simulink model "mVariantSubsystemConfig"  (R2019b)
settings: Solver=VariableStepAuto  StartTime=0.0  StopTime=10.0  RelTol=1e-3
settings Model: Creator=9bt  LastModifiedBy=4qz

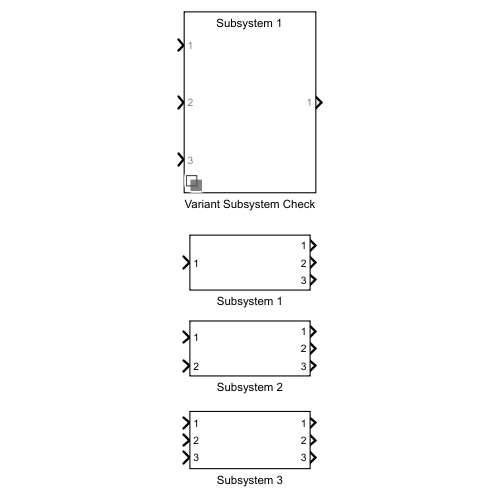
[thumbnail: Simulink's stored preview of the top-level diagram]
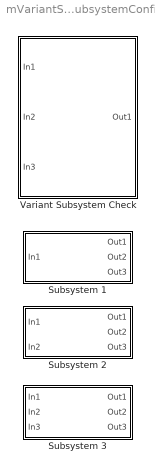
== system mVariantSubsystemConfig ==
  Subsystem 1 : Subsystem  VariantControl=Choice_1
  Subsystem 2 : Subsystem  VariantControl=Choice_2
  Subsystem 3 : Subsystem  VariantControl=Choice_3
  Variant Subsystem Check : Subsystem  Variant=on  VariantControlMode=label  LabelModeActiveChoice=Choice_1

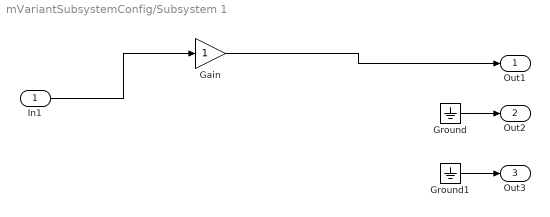
== system mVariantSubsystemConfig/Subsystem 1 ==
  In1 : Inport
  Gain : Gain
  Ground : Ground
  Ground1 : Ground
  Out1 : Outport
  Out2 : Outport  Port=2
  Out3 : Outport  Port=3
  wires:
  In1/1 -> Gain/1
  Gain/1 -> Out1/1
  Ground/1 -> Out2/1
  Ground1/1 -> Out3/1

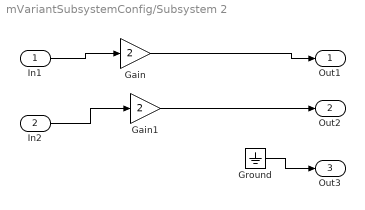
== system mVariantSubsystemConfig/Subsystem 2 ==
  In1 : Inport
  In2 : Inport  Port=2
  Gain : Gain  Gain=2
  Gain1 : Gain  Gain=2
  Ground : Ground
  Out1 : Outport
  Out2 : Outport  Port=2
  Out3 : Outport  Port=3
  wires:
  Gain1/1 -> Out2/1
  Gain/1 -> Out1/1
  In1/1 -> Gain/1
  In2/1 -> Gain1/1
  Ground/1 -> Out3/1

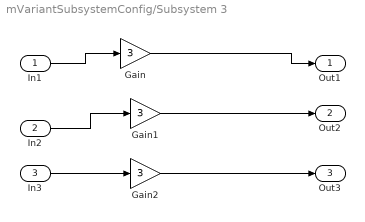
== system mVariantSubsystemConfig/Subsystem 3 ==
  In1 : Inport
  In2 : Inport  Port=2
  In3 : Inport  Port=3
  Gain : Gain  Gain=3
  Gain1 : Gain  Gain=3
  Gain2 : Gain  Gain=3
  Out1 : Outport
  Out2 : Outport  Port=2
  Out3 : Outport  Port=3
  wires:
  In2/1 -> Gain1/1
  Gain1/1 -> Out2/1
  Gain/1 -> Out1/1
  Gain2/1 -> Out3/1
  In1/1 -> Gain/1
  In3/1 -> Gain2/1

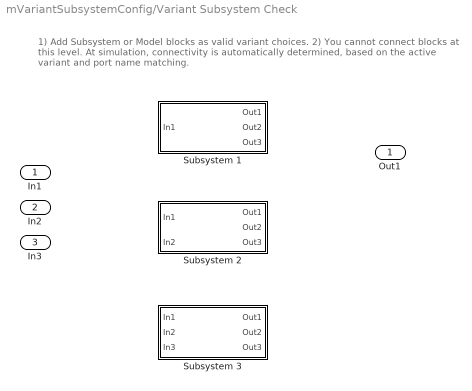
== system mVariantSubsystemConfig/Variant Subsystem Check ==
  note: 1) Add Subsystem or Model blocks as valid variant choices.
      | 2) You cannot connect blocks at this level. At simulation, connectivity is automatically
      | determined, based on the active variant and port name matching.
  In1 : Inport
  In2 : Inport  Port=2
  In3 : Inport  Port=3
  Subsystem 1 : Subsystem  VariantControl=Choice_1
  Subsystem 2 : Subsystem  VariantControl=Choice_2
  Subsystem 3 : Subsystem  VariantControl=Choice_3
  Out1 : Outport

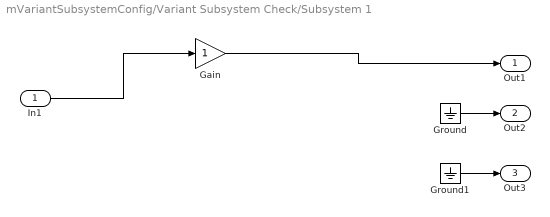
== system mVariantSubsystemConfig/Variant Subsystem Check/Subsystem 1 ==
  In1 : Inport
  Gain : Gain
  Ground : Ground
  Ground1 : Ground
  Out1 : Outport
  Out2 : Outport  Port=2
  Out3 : Outport  Port=3
  wires:
  In1/1 -> Gain/1
  Gain/1 -> Out1/1
  Ground/1 -> Out2/1
  Ground1/1 -> Out3/1

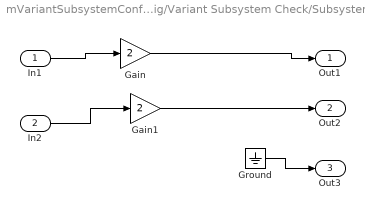
== system mVariantSubsystemConfig/Variant Subsystem Check/Subsystem 2 ==
  In1 : Inport
  In2 : Inport  Port=2
  Gain : Gain  Gain=2
  Gain1 : Gain  Gain=2
  Ground : Ground
  Out1 : Outport
  Out2 : Outport  Port=2
  Out3 : Outport  Port=3
  wires:
  Gain1/1 -> Out2/1
  Gain/1 -> Out1/1
  In1/1 -> Gain/1
  In2/1 -> Gain1/1
  Ground/1 -> Out3/1

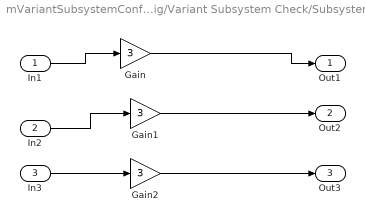
== system mVariantSubsystemConfig/Variant Subsystem Check/Subsystem 3 ==
  In1 : Inport
  In2 : Inport  Port=2
  In3 : Inport  Port=3
  Gain : Gain  Gain=3
  Gain1 : Gain  Gain=3
  Gain2 : Gain  Gain=3
  Out1 : Outport
  Out2 : Outport  Port=2
  Out3 : Outport  Port=3
  wires:
  In2/1 -> Gain1/1
  Gain1/1 -> Out2/1
  Gain/1 -> Out1/1
  Gain2/1 -> Out3/1
  In1/1 -> Gain/1
  In3/1 -> Gain2/1
